simulink model "Iphone_Send"  (R2016b)
settings: Solver=FixedStepAuto  StartTime=0.0  StopTime=10.0  RelTol=1e-3
libraries: ioslib x9
settings Model: Creator=Tonmai  LastModifiedBy=Tonmai
settings OptimizationCC: MaxStackSize=64
settings DebuggingCC: ParameterTunabilityLossMsg=error
settings HardwareCC: ProdBitPerPointer=32  ProdBitPerSizeT=32  ProdBitPerPtrDiffT=32  ProdLargestAtomicInteger=Long  ProdLargestAtomicFloat=Double  ProdWordSize=32  ProdHWDeviceType=ARM Compatible->ARM Cortex
settings RTWCC: SystemTargetFile=ert.tlc  HardwareBoard=Apple iOS Device  TLCOptions="-aInlineSetEventsForThisBaseRateFcn=TLC_FALSE -aSuppressMultiTaskScheduler=TLC_FALSE  -aRateBasedStepFcn=0"  TemplateMakefile=ert_default_tmf  Description=Embedded Coder  GenerateReport=on  Toolchain=Xcode iOS Project  IncludeHyperlinkInReport=on  LaunchReport=on  GenerateTraceInfo=on  GenerateTraceReport=on  GenerateTraceReportSl=on  GenerateTraceReportSf=on  GenerateTraceReportEml=on
settings CodeAppCC: ForceParamTrailComments=on  IgnoreCustomStorageClasses=off  OperatorAnnotations=on  SimulinkDataObjDesc=on  SFDataObjDesc=on  MATLABFcnDesc=on  InsertBlockDesc=on  MATLABSourceComments=on
settings ERTTargetCC: ExtModeMexArgs='0.0.0.0'

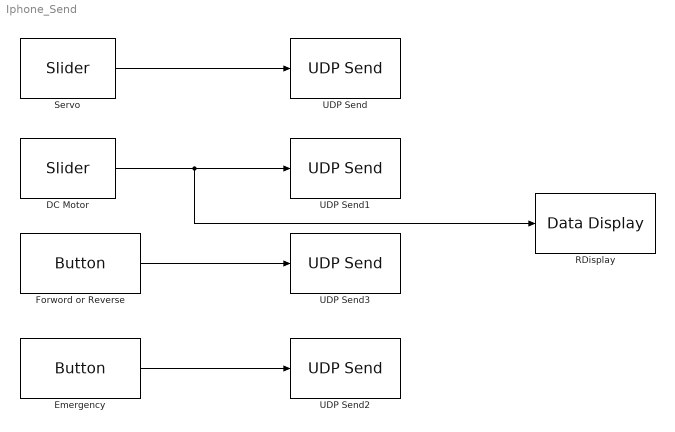
== system Iphone_Send ==
  DC Motor : ioslib/Slider  Min=0  Value=0  Max=40  Resolution=1  SliderId=Iphone_Send_DC_Motor  SampleTime=0.1  SimulateUsing=Code generation  blockPlatform=iOS
  Emergency : ioslib/Button  ButtonState=Not Pressed  ButtonId=Iphone_Send_Emergency  State=off  SimulateUsing=Code generation  SampleTime=0.1  BlockPlatform=iOS
  Forword or Reverse : ioslib/Button  ButtonState=Not Pressed  ButtonId=Iphone_Send_Forword_or_Reverse  State=off  SimulateUsing=Code generation  SampleTime=0.1  BlockPlatform=iOS
  RDisplay : ioslib/Data Display  DataDisplayId=Iphone_Send_RDisplay  Format=Float  Precision=6  SimulateUsing=Code generation  BlockPlatform=iOS
  Servo : ioslib/Slider  Min=40  Value=60  Max=100  Resolution=1  SliderId=Iphone_Send_Servo  SampleTime=0.1  SimulateUsing=Code generation  blockPlatform=iOS
  UDP Send : ioslib/UDP Send  remoteURL='10.26.4.178'  remotePort=26001  localURL='0.0.0.0'  localPortSource=Automatically determine  localPort=-1  sampletime=-1  blockPlatform=iOS  separateLengthPort=0
  UDP Send1 : ioslib/UDP Send  remoteURL='10.26.4.178'  remotePort=26002  localURL='0.0.0.0'  localPortSource=Automatically determine  localPort=-1  sampletime=-1  blockPlatform=iOS  separateLengthPort=0
  UDP Send2 : ioslib/UDP Send  remoteURL='10.26.4.178'  remotePort=26003  localURL='0.0.0.0'  localPortSource=Automatically determine  localPort=-1  sampletime=-1  blockPlatform=iOS  separateLengthPort=0
  UDP Send3 : ioslib/UDP Send  remoteURL='10.26.4.178'  remotePort=26004  localURL='0.0.0.0'  localPortSource=Automatically determine  localPort=-1  sampletime=-1  blockPlatform=iOS  separateLengthPort=0
  wires:
  Servo/1 -> UDP Send/1
  DC Motor/1 -> RDisplay/1, UDP Send1/1
  Emergency/1 -> UDP Send2/1
  Forword or Reverse/1 -> UDP Send3/1
